simulink model "prob5"  (Simulink 8.6)
settings: Solver=ode45  StartTime=0.0  StopTime=200  RelTol=1e-3
undefined symbols (not defined in the file or in its folder): altitude_hold_autopilot, P
settings Model: Creator=tmclain  LastModifiedBy=jae
settings DataIOCC: SignalLoggingSaveFormat=Dataset
settings DebuggingCC: FcnCallInpInsideContextMsg=EnableAllAsError
settings GRTTargetCC: CombineOutputUpdateFcns=on  GRTInterface=off

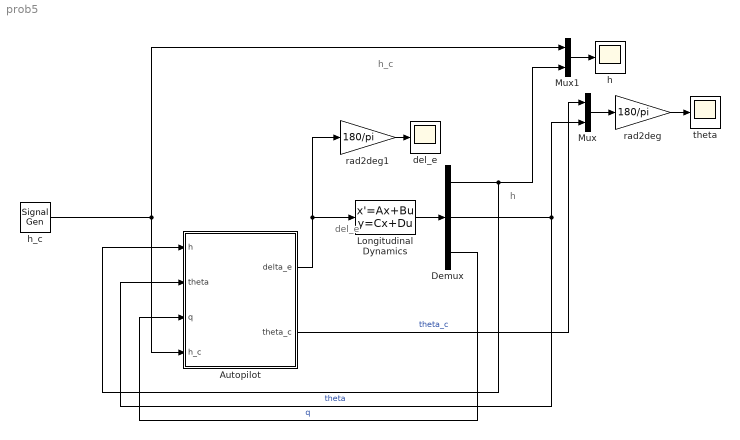
== system prob5 ==
  note: del_e
  note: h_c
  note: h
  Autopilot : Subsystem
  Demux : Demux  Outputs=3
  Longitudinal Dynamics : StateSpace  A=[-0.00643 0.0263 0 -32.2 0; -0.0941 -0.624 820 0 0; -0.000222 -0.00153 -0.668 0 0; 0 0 1 0 0; 0 -1 0 830 0]  B=[0; -32.7; -2.08; 0; 0]  C=[0 0 0 0 1; 0 0 0 1 0; 0 0 1 0 0]  D=[0; 0; 0]  X0=0
  Mux : Mux  Inputs=2
  Mux1 : Mux  Inputs=2
  del_e : Scope
  h : Scope
  h_c : SignalGenerator  WaveForm=square  Amplitude=100  Frequency=.0125
  rad2deg : Gain  Gain=180/pi
  rad2deg1 : Gain  Gain=180/pi
  theta : Scope
  wires:
  Longitudinal Dynamics/1 -> Demux/1
  Demux/1 -> Mux1/2, Autopilot/1(h)
  Demux/2 -> Autopilot/2(theta), Mux/2  "theta"
  Demux/3 -> Autopilot/3(q)  "q"
  rad2deg/1 -> theta/1
  Mux/1 -> rad2deg/1
  Mux1/1 -> h/1
  rad2deg1/1 -> del_e/1
  h_c/1 -> Autopilot/4(h_c), Mux1/1
  Autopilot/2(theta_c) -> Mux/1  "theta_c"
  Autopilot/1(delta_e) -> rad2deg1/1, Longitudinal Dynamics/1

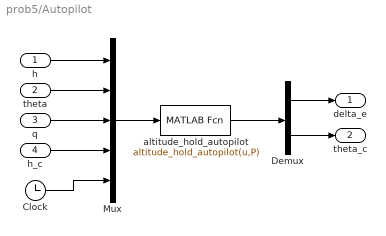
== system prob5/Autopilot ==
  h : Inport
  theta : Inport  Port=2
  q : Inport  Port=3
  h_c : Inport  Port=4
  Clock : Clock
  Demux : Demux  Outputs=2
  Mux : Mux  Inputs=5
  altitude_hold_autopilot : MATLABFcn  MATLABFcn=altitude_hold_autopilot(u,P)  OutputDimensions=2
  delta_e : Outport
  theta_c : Outport  Port=2
  wires:
  Mux/1 -> altitude_hold_autopilot/1
  altitude_hold_autopilot/1 -> Demux/1
  h/1 -> Mux/1
  theta/1 -> Mux/2
  q/1 -> Mux/3
  h_c/1 -> Mux/4
  Clock/1 -> Mux/5
  Demux/1 -> delta_e/1
  Demux/2 -> theta_c/1
